simulink library "lib_lowphy"  (R2023b)
settings: Solver=VariableStepAuto  StartTime=0.0  StopTime=10.0  RelTol=1e-3
undefined symbols (not defined in the file or in its folder): AdvDSPBChannelOutDisplay, AdvDSPBDMemDisplay, AdvDSPBInDisplay, AdvDSPBOutDisplay, dpoly, dspba, dspba_ChannelInVis, dspba_ChannelOutVis, dspba_internal_get_channel_ports, evalAionMaskParam, fft_tb_in, ifft_tb_in, latency, latencyCorrection, max_FFTStages, max_NSubcarriers, primtype, UseDontCare, value
libraries: DSPBAPrim x637, DSPBAControl x55, $bdroot x16, DSPBAModelBus x12, DSPBAUtilities x6, DSPBABase x5, DSPBAWaveformSynth x4, DspbAdvFftLibrary x3, DSPBAVectorUtil x2, DspbAdvVfftPrefix x1
(part 2 of 9)

== system lib_lowphy/FFT_S2B/SignalProcessing ==
  fft_v_in : Inport
  cin : Inport  Port=2
  din : Inport  Port=3
  sync : Inport  Port=4
  nsc : Inport  Port=5
  size : Inport  Port=6
  SFNin : Inport  Port=7
  fft_gain_re : Inport  Port=8
  fft_gain_im : Inport  Port=9
  hcs_bypass : Inport  Port=10
  fft_shift : Inport  Port=11
  DC_SC_EN : Inport  Port=12
  ripple_comp_en : Inport  Port=13
  rc_bw_sel : Inport  Port=14
  eAxc : Inport  Port=15
  sym_metadata : Inport  Port=16
  BRandSCSelect1 : Subsystem  Opaque=on  mask(DSP Builder Advanced FFT Blockset){N=dspb_fft_multichannel.FFTsize, subchannels=dspb_fft_multichannel.subchannels}
      mask prompts: N "FFT Size"; subchannels "Number of subchannels (must be a power of 2)"
      mask help: Performs bit reversal of incoming FFT frames.
      mask init:
      | block = gcb;
      | 
      | % Check that we have a legal size
      | M = ceil(log2(N));
      | if not(N == 2^M)
      |     error('%s: %d is not a power of 2', block, N);
      | end
      | 
      | % Check that we have a legal number os subchannels
      | subchannelbits = ceil(log2(subchannels));
      | if not(subchannels == 2^subchannelbits)
      |     error('%s: subchannels count %d is not a power of 2', block, N);
      | end
      | 
      | % The permutation reverses the order of the address bits
      | bitrevperm = [M-1:-1:0];
      | 
      | % Prefix permutaion with unchanging subchannel bits
      | bitrevperm = [0:subchannelbits-1,bitrevperm+subchannelbits];
      | 
      | if 1 < subchannels
      |     subchannelString = sprintf('%d subchannels',subchannels);
      | else
      |     subchannelString = '';
      | end
      mask Help: helpview(dspba.GetHelp('BitReverseCore'));
      mask Display:
      | color('w');
      | image('dspba_fft.jpg');
      | port_label('input',1,'v');
      | port_label('input',2,'c');
      | port_label('input',3,'x');
      | port_label('input',4,'size');
      | port_label('input',5,'NSubCarr');
      | port_label('output',1,'qv');
      | port_label('output',2,'qc');
      | port_label('output',3,'q');
      | text(0.25, 0.8, 'Bit Reversal');
      | text(0.2, 0.7, 'and SubCarrier');
      | text(0.3, 0.6, 'Selection');
      | text(0.20,0.35,subchannelString);
  HCShift : Subsystem
  RXGainComp : Subsystem
  RXScaling : Subsystem
  Terminator : Terminator
  Terminator1 : Terminator
  Terminator2 : Terminator
  VFFT_btb : Subsystem  AncestorBlock=DspbAdvVfftPrefix/VFFT_btb  Opaque=on  mask{IFFT=dspb_fft_multichannel.IFFT, subchannels=dspb_fft_multichannel.subchannels, br_in=false, maxSize=dspb_fft_multichannel.maxsize, minSize=dspb_fft_multichannel.minsize, in_type=dspb_fft_multichannel.InputType, type_strings=dspba.fft.full_wordgrowth(true,false,11,fixdt(1,16,15),fixdt(1,18,17)), faithful=true}
      mask prompts: subchannels "Number of interleaved subchannels (must be a power of 2)"; br_in "Bit-reversed input"; maxSize "maxSize, where the (I)FFT has at most 2^maxSize points"; minSize "minSize, where the (I)FFT has at least 2^minSize points"; in_type "Input type"; type_strings "Twiddle/pruning specification"; faithful "Use faithful rounding"
      mask init:
      | block = gcb;
      | 
      | % Check that we have a legal number of subchannels
      | subchannelbits = ceil(log2(subchannels));
      | if not(subchannels == 2^subchannelbits)
      |     error('%s: subchannels count %d is not a power of 2', block, subchannels);
      | end
      | 
      | if IFFT
      |     FFTstring = 'IFFT';
      | else
      |     FFTstring = 'FFT';
      | end
      | 
      | if br_in
      |     directionString = 'BR->NAT';
      | else
      |     directionString = 'NAT->BR';
      | end
      | 
      | if 1 < subchannels
      |     subchannelString = sprintf('%d subchannels',subchannels);
      | else
      |     subchannelString = '';
      | end
      | 
      | % Largest number going into the VPD/VPM control inputs
      | maxBlocksizeBits = maxSize + subchannelbits;
      | 
      | % The width of the datapath needed to hold this number
      | adderWidth = ceil(log2(maxBlocksizeBits+1));
      mask Help: helpview(dspba.GetHelp('fft'));
      mask Display:
      | color('w');
      | image('dspba_fft.jpg');
      | port_label('input',1,'v');
      | port_label('input',2,'c');
      | port_label('input',3,'sop');
      | port_label('input',4,'size');
      | port_label('input',5,'d');
      | port_label('input',6,'nsc');
      | port_label('output',1,'qv');
      | port_label('output',2,'qc');
      | port_label('output',3,'qsop');
      | port_label('output',4,'qeop');
      | port_label('output',5,'qsize');
      | port_label('output',6,'q');
      | %text(0.25,0.75,sprintf('Cyclic Prefix'));
      | text(0.30,0.65,sprintf('V%s Core',FFTstring));
      | text(0.35,0.55,sprintf('2^{%d} to 2^{%d}',minSize,maxSize),'texmode','on');
      | text(0.30,0.45,directionString);
      | text(0.20,0.30,subchannelString);
      | text(0.25,0.20,sprintf('Back-To-Back'));
  rxnat_vout : Outport
  rxnat_chout : Outport  Port=2
  rxnat_dout : Outport  Port=3
  rx_time_out : Outport  Port=4
  td_fft_in_v : Outport  Port=5
  td_fft_in_ch : Outport  Port=6
  td_fft_in_d : Outport  Port=7
  nsc_out : Outport  Port=8
  size_out : Outport  Port=9
  td_time_out : Outport  Port=10
  fd_v : Outport  Port=11
  fd_c : Outport  Port=12
  fd_q : Outport  Port=13
  eAxC : Outport  Port=14
  metadata_sym_out : Outport  Port=15
  wires:
  BRandSCSelect1/6(eAxC_out) -> eAxC/1
  BRandSCSelect1/5(time_out) -> rx_time_out/1
  BRandSCSelect1/7(meatadata_sym_out) -> metadata_sym_out/1
  BRandSCSelect1/4(qsizeout) -> Terminator2/1
  BRandSCSelect1/1(qv) -> rxnat_vout/1  "rx_v_out"
  rc_bw_sel/1 -> BRandSCSelect1/9(rc_bw_sel)
  RXScaling/5(nsc_out) -> BRandSCSelect1/5(NSubCarr)
  ripple_comp_en/1 -> BRandSCSelect1/8(ripple_comp_en)
  RXScaling/4(size_out) -> BRandSCSelect1/4(FFTSize)
  RXScaling/3(dout) -> BRandSCSelect1/3(x), fd_q/1
  RXScaling/2(chout) -> fd_c/1, BRandSCSelect1/2(c)
  fft_shift/1 -> RXScaling/6(fft_shift)
  VFFT_btb/10(metadata_sym) -> RXScaling/9(sym_metadata)
  VFFT_btb/2(qc) -> RXScaling/2(chin)
  size/1 -> HCShift/5(size)
  RXGainComp/5(size_out) -> VFFT_btb/6(size), size_out/1
  HCShift/1(vout) -> RXGainComp/1(vin)
  RXScaling/1(vout) -> BRandSCSelect1/1(v), fd_v/1
  VFFT_btb/7(qnsc) -> RXScaling/5(nsc)
  HCShift/3(dout) -> RXGainComp/3(din)
  din/1 -> HCShift/3(din)
  hcs_bypass/1 -> HCShift/7(hcs_bypass)
  HCShift/6(SFNout) -> RXGainComp/8(time_in)
  RXGainComp/1(vout) -> VFFT_btb/1(v), VFFT_btb/3(sop), td_fft_in_v/1
  SFNin/1 -> HCShift/8(SFNin)
  VFFT_btb/1(qv) -> RXScaling/1(vin)
  BRandSCSelect1/2(qc) -> rxnat_chout/1
  VFFT_btb/3(qsop) -> Terminator/1
  sym_metadata/1 -> HCShift/10(sym_metadata)
  VFFT_btb/9(eAxC) -> RXScaling/8(eAxC)
  VFFT_btb/5(qsize) -> RXScaling/3(size)
  eAxc/1 -> HCShift/9(eAxC)
  nsc/1 -> HCShift/6(nsc)
  cin/1 -> HCShift/2(cin)
  RXScaling/7(eAxCout) -> BRandSCSelect1/10(eAxC)
  VFFT_btb/6(q) -> RXScaling/4(din)
  fft_v_in/1 -> HCShift/1(vin)
  RXGainComp/3(dout) -> td_fft_in_d/1, VFFT_btb/4(d)
  DC_SC_EN/1 -> BRandSCSelect1/7(DC_SC_EN)
  HCShift/2(cout) -> RXGainComp/2(chin)
  HCShift/4(nsc_out) -> RXGainComp/4(nsc)
  RXScaling/6(time_out) -> BRandSCSelect1/6(time_in)
  sync/1 -> HCShift/4(sync)
  HCShift/5(size_out) -> RXGainComp/5(size)
  RXGainComp/2(chout) -> td_fft_in_ch/1, VFFT_btb/2(c)
  VFFT_btb/8(time_out) -> RXScaling/7(time_in)
  RXGainComp/6(time_out) -> td_time_out/1, VFFT_btb/7(time_in)
  fft_gain_re/1 -> RXGainComp/6(fft_gain_re)
  HCShift/7(eAxC_out) -> RXGainComp/9(eAxC)
  HCShift/8(sym_metadataout) -> RXGainComp/10(sym_metadata)
  fft_gain_im/1 -> RXGainComp/7(fft_gain_im)
  BRandSCSelect1/3(q) -> rxnat_dout/1
  RXScaling/8(sym_metadataout) -> BRandSCSelect1/11(metadata_in)
  RXGainComp/7(eAxC_out) -> VFFT_btb/8(eAxC_no)
  VFFT_btb/4(qeop) -> Terminator1/1
  RXGainComp/4(nsc_out) -> nsc_out/1, VFFT_btb/5(nsc)
  RXGainComp/8(sym_metadata_out) -> VFFT_btb/9(sym_metadata)

== system lib_lowphy/PhaseCompensation/ComplexMixer ==
  note: mixer
  din1 : Inport
  vin : Inport  Port=2
  cin : Inport  Port=3
  sin : Inport  Port=4
  cos : Inport  Port=5
  Add : DSPBAPrim/Add  primtype=add  nInputs=evalAionMaskParam(gcb,'value',1)  nOutputs=1  omode=Inherit via internal rule with word growth  otype=sfix(16)  scale=2^-15  rndmethod=Unbiased  factor=1  satmethod=Symmetric  shift_vec=[0 1 2 -1]  value=2  inPortNames=[' '; ' ';]  outPortNames=[' ']  dspbaimage=dspba_prim.svg  text=fprintf('+');  style=Optimised  visibilities=1032+2^17+2^18+2^19  genFPC=off  floatRounding=correct  advOptions=[]  version=20211007
  Complex to Real-Imag1 : ComplexToRealImag
  ComplexMixer : DSPBAWaveformSynth/ComplexMixer  nInputRate=dspb_ifft_multichannel.ClockRate  nchan=1  nfreq=1  latency=6  simulationMode=Use Global Value  version=20090407
      settings: AttributesFormatString=%<latency>
  Const1 : DSPBAPrim/Const  primtype=const  nInputs=0  nOutputs=1  omode=Inherit via back propagation  otype=ufix(8)  scale=2^0  rndmethod=Unbiased  factor=1  satmethod=Symmetric  shift_vec=[0 1 2 -1]  value=1  inPortNames=['+'; '+';]  outPortNames=[' ']  dspbaimage=dspba_prim.svg  text=fprintf('%s', num2str(value));  style=Optimised  visibilities=8 + 1024  floatPrecision=float32_m23  warnSaturation=on  version=20211007  SampleTime=inf
  Mult : DSPBAPrim/Mult  primtype=mult  nInputs=2  nOutputs=1  omode=Inherit via internal rule  otype=sfix(16)  scale=2^-15  rndmethod=Unbiased  factor=1  satmethod=Symmetric  shift_vec=[0 1 2 -1]  value=0  inPortNames=[' '; ' ';]  outPortNames=[' ']  dspbaimage=dspba_prim.svg  text=fprintf('X');  style=Optimised  visibilities=8+2^18+2^19  floatPrecision=float32_m23  floatRounding=correct  advOptions=[]  version=20211007
  Mult1 : DSPBAPrim/Mult  primtype=mult  nInputs=2  nOutputs=1  omode=Inherit via internal rule  otype=sfix(16)  scale=2^-15  rndmethod=Unbiased  factor=1  satmethod=Symmetric  shift_vec=[0 1 2 -1]  value=0  inPortNames=[' '; ' ';]  outPortNames=[' ']  dspbaimage=dspba_prim.svg  text=fprintf('X');  style=Optimised  visibilities=8+2^18+2^19  floatPrecision=float32_m23  floatRounding=correct  advOptions=[]  version=20211007
  Real-Imag to Complex : RealImagToComplex
  Scalei : DSPBABase/Scale  otype=sfix(16)  scale=Op_frac_scaling  rndmethod=Biased  factor=1  satmethod=None  shift_vec=0  latency=1  simulationMode=Use Global Value  version=20130807
      settings: AttributesFormatString=%<latency>
  Scaleq : DSPBABase/Scale  otype=sfix(16)  scale=Op_frac_scaling  rndmethod=Biased  factor=1  satmethod=None  shift_vec=0  latency=1  simulationMode=Use Global Value  version=20130807
      settings: AttributesFormatString=%<latency>
  Scope : Scope
  Terminator{4..7} (4 alike) : Terminator
  dout1 : Outport
  vout : Outport  Port=2
  cout : Outport  Port=3
  wires:
  din1/1 -> Complex to Real-Imag1/1
  Scaleq/1 -> Real-Imag to Complex/2
  ComplexMixer/3 -> Scaleq/2, Scalei/2
  Scalei/1 -> Real-Imag to Complex/1
  Const1/1 -> Scaleq/4, Scalei/4
  Scaleq/3 -> Terminator7/1
  ComplexMixer/2 -> Scaleq/1
  Scaleq/2 -> Terminator6/1
  ComplexMixer/4 -> Scaleq/3, Scalei/3
  Complex to Real-Imag1/1 -> ComplexMixer/1
  Scalei/4 -> Terminator5/1
  Scaleq/4 -> Terminator4/1
  Complex to Real-Imag1/2 -> ComplexMixer/2
  ComplexMixer/1 -> Scalei/1
  Real-Imag to Complex/1 -> dout1/1
  sin/1 -> Mult/2, Mult/1, ComplexMixer/5
  vin/1 -> ComplexMixer/3
  cin/1 -> ComplexMixer/4
  cos/1 -> Mult1/2, Mult1/1, ComplexMixer/6
  Scalei/2 -> vout/1
  Scalei/3 -> cout/1
  Mult/1 -> Add/1
  Mult1/1 -> Add/2
  Add/1 -> Scope/1

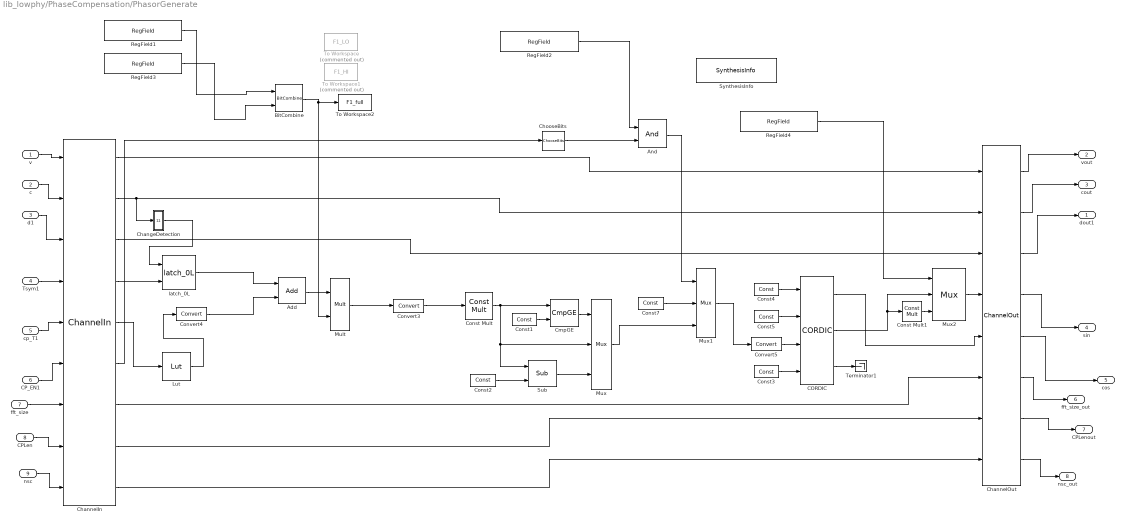
== system lib_lowphy/PhaseCompensation/PhasorGenerate ==
  v : Inport
  c : Inport  Port=2
  d1 : Inport  Port=3
  Tsym1 : Inport  Port=4
  cp_T1 : Inport  Port=5
  CP_EN1 : Inport  Port=6
  fft_size : Inport  Port=7
  CPLen : Inport  Port=8
  nsc : Inport  Port=9
  Add : DSPBAPrim/Add  primtype=add  nInputs=evalAionMaskParam(gcb,'value',1)  nOutputs=1  omode=Inherit via internal rule  otype=sfix(16)  scale=2^-15  rndmethod=Unbiased  factor=1  satmethod=Symmetric  shift_vec=[0 1 2 -1]  value=2  inPortNames=[' '; ' ';]  outPortNames=[' ']  dspbaimage=dspba_prim.svg  text=fprintf('+');  style=Optimised  visibilities=1032+2^17+2^18+2^19  genFPC=off  floatRounding=correct  advOptions=[]  version=20211007
  And : DSPBAPrim/And  primtype=and  nInputs=2  nOutputs=1  omode=Inherit via internal rule  otype=sfix(16)  scale=2^-15  rndmethod=Unbiased  factor=1  satmethod=Symmetric  shift_vec=[0 1 2 -1]  value=0  inPortNames=[' '; ' '; ' '; ' '; ' '; ' '; ' '; ' '; ' '; ' '; ' '; ' '; ' '; ' '; ' '; ' '; ]  outPortNames=[' ']  dspbaimage=dspba_prim.svg  text=fprintf('&');  style=Optimised  visibilities=8+2  version=20211007
  BitCombine : DSPBAPrim/BitCombine  primtype=bitcombine  nInputs=2  nOutputs=1  omode=Specify via dialog  otype=ufix(64)  scale=2^-56  rndmethod=Unbiased  factor=1  satmethod=Symmetric  shift_vec=[0 1 2 -1]  value=0  inPortNames=['l'; 'h';]  outPortNames=[' ']  dspbaimage=dspba_prim.svg  text=fprintf('[h,l]');  style=Optimised  visibilities=8+2  version=20211007
  CORDIC : DSPBAPrim/CORDIC  primtype=cordic  nInputs=4  nOutputs=3  omode=Inherit via internal rule  otype=sfix(16)  scale=2^-15  rndmethod=Unbiased  factor=1  satmethod=Symmetric  shift_vec=[0 1 2 -1]  value=0  inPortNames=['x'; 'y'; 'p'; 'v']  outPortNames=['x'; 'y'; 'p']  dspbaimage=dspba_prim_tall.svg  text=fprintf('cordic');  style=Optimised  visibilities=8  version=20211007
  ChangeDetection : Subsystem
  ChannelIn : DSPBAPrim/ChannelIn  primtype=channelin  nInputs=dspba_internal_get_channel_ports(gcb)  nOutputs=dspba_internal_get_channel_ports(gcb)  omode=Inherit via internal rule  otype=sfix(16)  scale=2^-15  rndmethod=Unbiased  factor=1  satmethod=Symmetric  shift_vec=[0 1 2 -1]  value=7  inPortNames=['v'; 'c'; '0'; '1'; '2'; '3'; '4'; '5'; '6'; '7'; '8'; '9'; 'A'; 'B'; 'D'; 'E'; 'F'; 'G'; 'H'; 'I'; 'J'; 'K'; 'L'; 'M'; 'N'; 'O'; 'P'; 'Q'; 'R'; 'S'; 'T'; 'U'; 'W'; 'X'; 'Y'; 'Z']  outPortNames=['v'; 'c'; '0'; '1'; '2'; '3'; '4'; '5'; '6'; '7'; '8'; '9'; 'A'; 'B'; 'D'; 'E'; 'F'; 'G'; 'H'; 'I'; 'J'; 'K'; 'L'; 'M'; 'N'; 'O'; 'P'; 'Q'; 'R'; 'S'; 'T'; 'U'; 'W'; 'X'; 'Y'; 'Z']  dspbaimage=dspba_prim_channel_tall.svg  text=fprintf('In');  style=Optimised  dataSignals=7  foldingEnabled=off  channels=1  sampleRate=200  packetBeginPresent=off  packetBeginEnabled=off  visibilities=dspba_ChannelInVis(gcb)  latencyCorrection=0  scheduleOrigin=on  version=20211214
  ChannelOut : DSPBAPrim/ChannelOut  primtype=channelout  nInputs=dspba_internal_get_channel_ports(gcb)  nOutputs=dspba_internal_get_channel_ports(gcb)  omode=Inherit via internal rule  otype=sfix(16)  scale=2^-15  rndmethod=Unbiased  factor=1  satmethod=Symmetric  shift_vec=[0 1 2 -1]  value=6  inPortNames=['v'; 'c'; '0'; '1'; '2'; '3'; '4'; '5'; '6'; '7'; '8'; '9'; 'A'; 'B'; 'D'; 'E'; 'F'; 'G'; 'H'; 'I'; 'J'; 'K'; 'L'; 'M'; 'N'; 'O'; 'P'; 'Q'; 'R'; 'S'; 'T'; 'U'; 'W'; 'X'; 'Y'; 'Z']  outPortNames=['v'; 'c'; '0'; '1'; '2'; '3'; '4'; '5'; '6'; '7'; '8'; '9'; 'A'; 'B'; 'D'; 'E'; 'F'; 'G'; 'H'; 'I'; 'J'; 'K'; 'L'; 'M'; 'N'; 'O'; 'P'; 'Q'; 'R'; 'S'; 'T'; 'U'; 'W'; 'X'; 'Y'; 'Z']  dspbaimage=dspba_prim_channel_tall.svg  text=fprintf('Out%s', AdvDSPBChannelOutDisplay(latency));  style=Optimised  dataSignals=6  foldingEnabled=off  channels=1  sampleRate=200  packetBeginPresent=off  packetBeginEnabled=off  visibilities=dspba_ChannelOutVis(gcb)  latency=38  latencyCorrection=0  version=20211214
  ChooseBits : DSPBAPrim/ChooseBits  primtype=choosebits  nInputs=1  nOutputs=1  omode=Inherit via internal rule  otype=fixdt(0,1,1)  scale=1  rndmethod=Unbiased  factor=1  satmethod=Symmetric  shift_vec=[0 1 2 -1]  value=[0]  inPortNames=[' '; ' ';]  outPortNames=[' ']  dspbaimage=dspba_prim.svg  text=fprintf('%s',dspba.perm2str(value));  style=Optimised  visibilities=1024  version=20211007
  CmpGE : DSPBAPrim/CmpGE  primtype=cmpgte  nInputs=2  nOutputs=1  omode=boolean  otype=sfix(16)  scale=2^-15  rndmethod=Unbiased  factor=1  satmethod=Symmetric  shift_vec=[0 1 2 -1]  value=0  inPortNames=['a'; 'b';]  outPortNames=[' ']  dspbaimage=dspba_prim.svg  text=fprintf('a>=b');  style=Optimised  visibilities=0  advOptions=[]  version=20211007
  Const Mult : DSPBAPrim/Const Mult  primtype=constmult  nInputs=1  nOutputs=1  omode=Specify via dialog  otype=sfix(16)  scale=2^-12  rndmethod=Unbiased  factor=1  satmethod=Symmetric  shift_vec=[0 1 2 -1]  value=2*pi  inPortNames=[' '; ' ';]  outPortNames=[' ']  dspbaimage=dspba_prim.svg  text=fprintf('cx');  style=Optimised  visibilities=8+2^10+2^17+2^18  floatRounding=correct  advOptions=[]  version=20211007
  Const Mult1 : DSPBAPrim/Const Mult  primtype=constmult  nInputs=1  nOutputs=1  omode=Specify via dialog  otype=sfix(16)  scale=2^-12  rndmethod=Unbiased  factor=1  satmethod=Symmetric  shift_vec=[0 1 2 -1]  value=-1  inPortNames=[' '; ' ';]  outPortNames=[' ']  dspbaimage=dspba_prim.svg  text=fprintf('cx');  style=Optimised  visibilities=8+2^10+2^17+2^18  floatRounding=correct  advOptions=[]  version=20211007
  Const1 : DSPBAPrim/Const  primtype=const  nInputs=0  nOutputs=1  omode=Specify via dialog  otype=sfix(16)  scale=2^-12  rndmethod=Unbiased  factor=1  satmethod=Symmetric  shift_vec=[0 1 2 -1]  value=pi  inPortNames=['+'; '+';]  outPortNames=[' ']  dspbaimage=dspba_prim.svg  text=fprintf('%s', num2str(value));  style=Optimised  visibilities=8 + 1024  floatPrecision=float32_m23  warnSaturation=on  version=20211007  SampleTime=inf
  Const2 : DSPBAPrim/Const  primtype=const  nInputs=0  nOutputs=1  omode=Specify via dialog  otype=sfix(16)  scale=2^-12  rndmethod=Unbiased  factor=1  satmethod=Symmetric  shift_vec=[0 1 2 -1]  value=2*pi  inPortNames=['+'; '+';]  outPortNames=[' ']  dspbaimage=dspba_prim.svg  text=fprintf('%s', num2str(value));  style=Optimised  visibilities=8 + 1024  floatPrecision=float32_m23  warnSaturation=on  version=20211007  SampleTime=inf
  Const3 : DSPBAPrim/Const  primtype=const  nInputs=0  nOutputs=1  omode=boolean  otype=sfix(16)  scale=2^-12  rndmethod=Unbiased  factor=1  satmethod=Symmetric  shift_vec=[0 1 2 -1]  value=0  inPortNames=['+'; '+';]  outPortNames=[' ']  dspbaimage=dspba_prim.svg  text=fprintf('%s', num2str(value));  style=Optimised  visibilities=8 + 1024  floatPrecision=float32_m23  warnSaturation=on  version=20211007  SampleTime=inf
  Const4 : DSPBAPrim/Const  primtype=const  nInputs=0  nOutputs=1  omode=Specify via dialog  otype=sfix(16)  scale=2^-15  rndmethod=Unbiased  factor=1  satmethod=Symmetric  shift_vec=[0 1 2 -1]  value=1/cordic_gain  inPortNames=['+'; '+';]  outPortNames=[' ']  dspbaimage=dspba_prim.svg  text=fprintf('%s', num2str(value));  style=Optimised  visibilities=8 + 1024  floatPrecision=float32_m23  warnSaturation=on  version=20211007  SampleTime=inf
  Const5 : DSPBAPrim/Const  primtype=const  nInputs=0  nOutputs=1  omode=Specify via dialog  otype=sfix(16)  scale=2^-15  rndmethod=Unbiased  factor=1  satmethod=Symmetric  shift_vec=[0 1 2 -1]  value=0  inPortNames=['+'; '+';]  outPortNames=[' ']  dspbaimage=dspba_prim.svg  text=fprintf('%s', num2str(value));  style=Optimised  visibilities=8 + 1024  floatPrecision=float32_m23  warnSaturation=on  version=20211007  SampleTime=inf
  Const7 : DSPBAPrim/Const  primtype=const  nInputs=0  nOutputs=1  omode=Specify via dialog  otype=sfix(16)  scale=2^-15  rndmethod=Unbiased  factor=1  satmethod=Symmetric  shift_vec=[0 1 2 -1]  value=0  inPortNames=['+'; '+';]  outPortNames=[' ']  dspbaimage=dspba_prim.svg  text=fprintf('%s', num2str(value));  style=Optimised  visibilities=8 + 1024  floatPrecision=float32_m23  warnSaturation=on  version=20211007  SampleTime=inf
  Convert3 : DSPBAPrim/Convert  primtype=convert  nInputs=1  nOutputs=1  omode=Specify via dialog  otype=ufix(16)  scale=2^-16  rndmethod=Biased  factor=1  satmethod=None  shift_vec=[0 1 2 -1]  value=round([0:255]/17)  inPortNames=[' '; ' ';]  outPortNames=[' '; 'c']  dspbaimage=dspba_prim_wide.svg  text=fprintf('convert');  style=Optimised  visibilities=8+64+256+2^17  clipdetect=off  floatPrecision=float32_m23  advOptions=[]  version=20211007
  Convert4 : DSPBAPrim/Convert  primtype=convert  nInputs=1  nOutputs=1  omode=Specify via dialog  otype=ufix(32)  scale=2^-18  rndmethod=Biased  factor=1  satmethod=None  shift_vec=[0 1 2 -1]  value=round([0:255]/17)  inPortNames=[' '; ' ';]  outPortNames=[' '; 'c']  dspbaimage=dspba_prim_wide.svg  text=fprintf('convert');  style=Optimised  visibilities=8+64+256+2^17  clipdetect=off  floatPrecision=float32_m23  advOptions=[]  version=20211007
  Convert5 : DSPBAPrim/Convert  primtype=convert  nInputs=1  nOutputs=1  omode=Specify via dialog  otype=sfix(16)  scale=2^-13  rndmethod=Biased  factor=1  satmethod=None  shift_vec=[0 1 2 -1]  value=round([0:255]/17)  inPortNames=[' '; ' ';]  outPortNames=[' '; 'c']  dspbaimage=dspba_prim_wide.svg  text=fprintf('convert');  style=Optimised  visibilities=8+64+256+2^17  clipdetect=off  floatPrecision=float32_m23  advOptions=[]  version=20211007
  Lut : DSPBAPrim/Lut  primtype=lut  nInputs=1  nOutputs=1  omode=Inherit via internal rule  otype=sfix(16)  scale=2^-15  rndmethod=Unbiased  factor=1  satmethod=Symmetric  shift_vec=[0 1 2 -1]  value=CPSample_Vector_LUT  inPortNames=[' '; ' ';]  outPortNames=[' ']  dspbaimage=dspba_prim.svg  text=fprintf('LUT');  style=Optimised  visibilities=8 + 1024  floatPrecision=float32_m23  version=20211007
  Mult : DSPBAPrim/Mult  primtype=mult  nInputs=2  nOutputs=1  omode=Inherit via internal rule  otype=sfix(16)  scale=2^-15  rndmethod=Unbiased  factor=1  satmethod=Symmetric  shift_vec=[0 1 2 -1]  value=0  inPortNames=[' '; ' ';]  outPortNames=[' ']  dspbaimage=dspba_prim.svg  text=fprintf('X');  style=Optimised  visibilities=8+2^18+2^19  floatPrecision=float64_m52  floatRounding=correct  advOptions=[]  version=20211007
  Mux : DSPBAPrim/Mux  primtype=mux  nInputs=evalAionMaskParam(gcb,'value',1)+1  nOutputs=1  omode=Inherit via internal rule  otype=sfix(16)  scale=2^-15  rndmethod=Unbiased  factor=1  satmethod=Symmetric  shift_vec=[0 1 2 -1]  value=2  inPortNames=['s '; 'd0'; 'd1'; 'd2'; 'd3'; 'd4'; 'd5'; 'd6'; 'd7'; 'd8'; 'd9';]  outPortNames=[' ']  dspbaimage=dspba_prim_tall.svg  text=fprintf('%s', primtype);  style=Optimised  visibilities=1032  version=20211007
  Mux1 : DSPBAPrim/Mux  primtype=mux  nInputs=evalAionMaskParam(gcb,'value',1)+1  nOutputs=1  omode=Inherit via internal rule  otype=sfix(16)  scale=2^-15  rndmethod=Unbiased  factor=1  satmethod=Symmetric  shift_vec=[0 1 2 -1]  value=2  inPortNames=['s '; 'd0'; 'd1'; 'd2'; 'd3'; 'd4'; 'd5'; 'd6'; 'd7'; 'd8'; 'd9';]  outPortNames=[' ']  dspbaimage=dspba_prim_tall.svg  text=fprintf('%s', primtype);  style=Optimised  visibilities=1032  version=20211007
  Mux2 : DSPBAPrim/Mux  primtype=mux  nInputs=evalAionMaskParam(gcb,'value',1)+1  nOutputs=1  omode=Specify via dialog  otype=sfix(18)  scale=2^-15  rndmethod=Unbiased  factor=1  satmethod=Symmetric  shift_vec=[0 1 2 -1]  value=2  inPortNames=['s '; 'd0'; 'd1'; 'd2'; 'd3'; 'd4'; 'd5'; 'd6'; 'd7'; 'd8'; 'd9';]  outPortNames=[' ']  dspbaimage=dspba_prim_tall.svg  text=fprintf('%s', primtype);  style=Optimised  visibilities=1032  version=20211007
  RegField1 : DSPBAModelBus/RegField  reg_name=MMoffset.F1_regLSB  reg_rwmode=Read/Write  reg_msb=31  reg_lsb=0  reg_mode=Specify via dialog  reg_type=ufix(32)  reg_scale=2^0  reg_init=F1_LSB  reg_desc=32 bit LSB of Carrier Center Frequency  reg_modal=off  reg_desc0=0  reg_desc1=0  reg_desc2=0  reg_desc3=0  reg_desc4=0  reg_desc5=0  reg_desc6=0  reg_desc7=0  reg_addr=0  SampleTime=-1  version=20090407
  RegField2 : DSPBAModelBus/RegField  reg_name=MMoffset.Enable_reg1  reg_rwmode=Read/Write  reg_msb=0  reg_lsb=0  reg_mode=Specify via dialog  reg_type=ufix(1)  reg_scale=2^0  reg_init=1  reg_desc=Enable/Disable Phase Compensation  reg_modal=off  reg_desc0=0  reg_desc1=0  reg_desc2=0  reg_desc3=0  reg_desc4=0  reg_desc5=0  reg_desc6=0  reg_desc7=0  reg_addr=2  SampleTime=-1  version=20090407
  RegField3 : DSPBAModelBus/RegField  reg_name=MMoffset.F1_regMSB  reg_rwmode=Read/Write  reg_msb=31  reg_lsb=0  reg_mode=Specify via dialog  reg_type=ufix(32)  reg_scale=2^0  reg_init=F1_MSB  reg_desc=32 bit MSB of Carrier Center Frequency  reg_modal=off  reg_desc0=0  reg_desc1=0  reg_desc2=0  reg_desc3=0  reg_desc4=0  reg_desc5=0  reg_desc6=0  reg_desc7=0  reg_addr=1  SampleTime=-1  version=20090407
  RegField4 : DSPBAModelBus/RegField  reg_name=MMoffset.PhaseGen_reg  reg_rwmode=Read/Write  reg_msb=0  reg_lsb=0  reg_mode=Specify via dialog  reg_type=ufix(1)  reg_scale=2^0  reg_init=PhaseGen_TXRX  reg_desc=Enable/Disable Phase Compensation  reg_modal=off  reg_desc0=0  reg_desc1=0  reg_desc2=0  reg_desc3=0  reg_desc4=0  reg_desc5=0  reg_desc6=0  reg_desc7=0  reg_addr=3  SampleTime=-1  version=20090407
  Sub : DSPBAPrim/Sub  primtype=sub  nInputs=2  nOutputs=1  omode=Inherit via internal rule with word growth  otype=sfix(16)  scale=2^-15  rndmethod=Unbiased  factor=1  satmethod=Symmetric  shift_vec=[0 1 2 -1]  value=0  inPortNames=['+'; '-';]  outPortNames=[' ']  dspbaimage=dspba_prim.svg  text=fprintf('-');  style=Optimised  visibilities=8+2^17+2^18  floatRounding=correct  advOptions=[]  version=20211007
  SynthesisInfo : DSPBAPrim/SynthesisInfo  primtype=synthinfo  nInputs=0  nOutputs=0  omode=Inherit via internal rule  otype=sfix(16)  scale=2^-15  rndmethod=Truncate  factor=1  satmethod=Symmetric  shift_vec=[0 1 2 -1]  value=99  inPortNames=[' '; ' ';]  outPortNames=[' ']  dspbaimage=dspba_prim_ctrl.jpg  text=fprintf('Style=%s', style);  style=Scheduled  visibilities=2^17+2^18+2^19+2^20+2^21+2^22+2^23+2^24  constraintPair=None  constraintRelation=>  constraintLimit=2  modelRefSign=+  modelRef=''  showSchedule=off  simulationMode=Use Global Value  resetMinimization=Conditional - On for ChannelIn/Out only  version=20220106
  Terminator1 : Terminator
  To Workspace : ToWorkspace  Commented=on  VariableName=F1_LO  SampleTime=-1
  To Workspace1 : ToWorkspace  Commented=on  VariableName=F1_HI  SampleTime=-1
  To Workspace2 : ToWorkspace  VariableName=F1_full  SampleTime=-1
  latch_0L : DSPBAControl/latch_0L
  dout1 : Outport
  vout : Outport  Port=2
  cout : Outport  Port=3
  sin : Outport  Port=4
  cos : Outport  Port=5
  fft_size_out : Outport  Port=6
  CPLenout : Outport  Port=7
  nsc_out : Outport  Port=8
  wires:
  c/1 -> ChannelIn/2
  ChannelIn/1 -> ChannelOut/1
  ChannelIn/2 -> ChangeDetection/1(In1), ChannelOut/2
  v/1 -> ChannelIn/1
  ChannelIn/3 -> ChannelOut/3
  d1/1 -> ChannelIn/3
  ChannelOut/1 -> vout/1
  ChannelOut/2 -> cout/1
  ChannelOut/3 -> dout1/1
  ChannelOut/4 -> sin/1
  ChannelIn/5 -> Lut/1
  Convert3/1 -> Const Mult/1
  Const Mult/1 -> Sub/1, Mux/2, CmpGE/1
  Const1/1 -> CmpGE/2
  CmpGE/1 -> Mux/1
  Sub/1 -> Mux/3
  Const2/1 -> Sub/2
  Const3/1 -> CORDIC/4
  Const4/1 -> CORDIC/1
  Const5/1 -> CORDIC/2
  CORDIC/3 -> Terminator1/1
  Convert5/1 -> CORDIC/3
  ChannelOut/5 -> cos/1
  RegField2/1 -> And/1
  Const7/1 -> Mux1/2
  CORDIC/1 -> ChannelOut/5
  Mux1/1 -> Convert5/1
  Lut/1 -> Convert4/1
  Mult/1 -> Convert3/1
  Mux/1 -> Mux1/3
  Add/1 -> Mult/1
  Convert4/1 -> Add/2
  ChannelIn/6 -> ChooseBits/1
  And/1 -> Mux1/1
  ChooseBits/1 -> And/2
  BitCombine/1 -> Mult/2, To Workspace2/1
  Tsym1/1 -> ChannelIn/4
  cp_T1/1 -> ChannelIn/5
  CP_EN1/1 -> ChannelIn/6
  RegField3/1 -> BitCombine/2
  RegField1/1 -> BitCombine/1
  fft_size/1 -> ChannelIn/7
  CPLen/1 -> ChannelIn/8
  nsc/1 -> ChannelIn/9
  ChannelOut/6 -> fft_size_out/1
  ChannelOut/7 -> CPLenout/1
  ChannelOut/8 -> nsc_out/1
  ChannelIn/7 -> ChannelOut/6
  ChannelIn/8 -> ChannelOut/7
  ChannelIn/9 -> ChannelOut/8
  latch_0L/1 -> Add/1
  ChangeDetection/1(Out1) -> latch_0L/1
  ChannelIn/4 -> latch_0L/2
  Mux2/1 -> ChannelOut/4
  CORDIC/2 -> Const Mult1/1, Mux2/2
  Const Mult1/1 -> Mux2/3
  RegField4/1 -> Mux2/1

== system lib_lowphy/PhaseCompensation_lite/ComplexMixer ==
  note: mixer
  din1 : Inport
  vin : Inport  Port=2
  cin : Inport  Port=3
  sin : Inport  Port=4
  cos : Inport  Port=5
  Add : DSPBAPrim/Add  primtype=add  nInputs=evalAionMaskParam(gcb,'value',1)  nOutputs=1  omode=Inherit via internal rule with word growth  otype=sfix(16)  scale=2^-15  rndmethod=Unbiased  factor=1  satmethod=Symmetric  shift_vec=[0 1 2 -1]  value=2  inPortNames=[' '; ' ';]  outPortNames=[' ']  dspbaimage=dspba_prim.svg  text=fprintf('+');  style=Optimised  visibilities=1032+2^17+2^18+2^19  genFPC=off  floatRounding=correct  advOptions=[]  version=20211007
  Complex to Real-Imag1 : ComplexToRealImag
  ComplexMixer : DSPBAWaveformSynth/ComplexMixer  nInputRate=dspb_ifft_multichannel.ClockRate  nchan=1  nfreq=1  latency=6  simulationMode=Use Global Value  version=20090407
      settings: AttributesFormatString=%<latency>
  Const1 : DSPBAPrim/Const  primtype=const  nInputs=0  nOutputs=1  omode=Inherit via back propagation  otype=ufix(8)  scale=2^0  rndmethod=Unbiased  factor=1  satmethod=Symmetric  shift_vec=[0 1 2 -1]  value=1  inPortNames=['+'; '+';]  outPortNames=[' ']  dspbaimage=dspba_prim.svg  text=fprintf('%s', num2str(value));  style=Optimised  visibilities=8 + 1024  floatPrecision=float32_m23  warnSaturation=on  version=20211007  SampleTime=inf
  Mult : DSPBAPrim/Mult  primtype=mult  nInputs=2  nOutputs=1  omode=Inherit via internal rule  otype=sfix(16)  scale=2^-15  rndmethod=Unbiased  factor=1  satmethod=Symmetric  shift_vec=[0 1 2 -1]  value=0  inPortNames=[' '; ' ';]  outPortNames=[' ']  dspbaimage=dspba_prim.svg  text=fprintf('X');  style=Optimised  visibilities=8+2^18+2^19  floatPrecision=float32_m23  floatRounding=correct  advOptions=[]  version=20211007
  Mult1 : DSPBAPrim/Mult  primtype=mult  nInputs=2  nOutputs=1  omode=Inherit via internal rule  otype=sfix(16)  scale=2^-15  rndmethod=Unbiased  factor=1  satmethod=Symmetric  shift_vec=[0 1 2 -1]  value=0  inPortNames=[' '; ' ';]  outPortNames=[' ']  dspbaimage=dspba_prim.svg  text=fprintf('X');  style=Optimised  visibilities=8+2^18+2^19  floatPrecision=float32_m23  floatRounding=correct  advOptions=[]  version=20211007
  Real-Imag to Complex : RealImagToComplex
  Scalei : DSPBABase/Scale  otype=sfix(16)  scale=Op_frac_scaling  rndmethod=Biased  factor=1  satmethod=None  shift_vec=0  latency=1  simulationMode=Use Global Value  version=20130807
      settings: AttributesFormatString=%<latency>
  Scaleq : DSPBABase/Scale  otype=sfix(16)  scale=Op_frac_scaling  rndmethod=Biased  factor=1  satmethod=None  shift_vec=0  latency=1  simulationMode=Use Global Value  version=20130807
      settings: AttributesFormatString=%<latency>
  Scope : Scope
  Terminator{4..7} (4 alike) : Terminator
  dout1 : Outport
  vout : Outport  Port=2
  cout : Outport  Port=3
  wires:
  din1/1 -> Complex to Real-Imag1/1
  Scaleq/1 -> Real-Imag to Complex/2
  ComplexMixer/3 -> Scaleq/2, Scalei/2
  Scalei/1 -> Real-Imag to Complex/1
  Const1/1 -> Scaleq/4, Scalei/4
  Scaleq/3 -> Terminator7/1
  ComplexMixer/2 -> Scaleq/1
  Scaleq/2 -> Terminator6/1
  ComplexMixer/4 -> Scaleq/3, Scalei/3
  Complex to Real-Imag1/1 -> ComplexMixer/1
  Scalei/4 -> Terminator5/1
  Scaleq/4 -> Terminator4/1
  Complex to Real-Imag1/2 -> ComplexMixer/2
  ComplexMixer/1 -> Scalei/1
  Real-Imag to Complex/1 -> dout1/1
  sin/1 -> Mult/2, Mult/1, ComplexMixer/5
  vin/1 -> ComplexMixer/3
  cin/1 -> ComplexMixer/4
  cos/1 -> Mult1/2, Mult1/1, ComplexMixer/6
  Scalei/2 -> vout/1
  Scalei/3 -> cout/1
  Mult/1 -> Add/1
  Mult1/1 -> Add/2
  Add/1 -> Scope/1

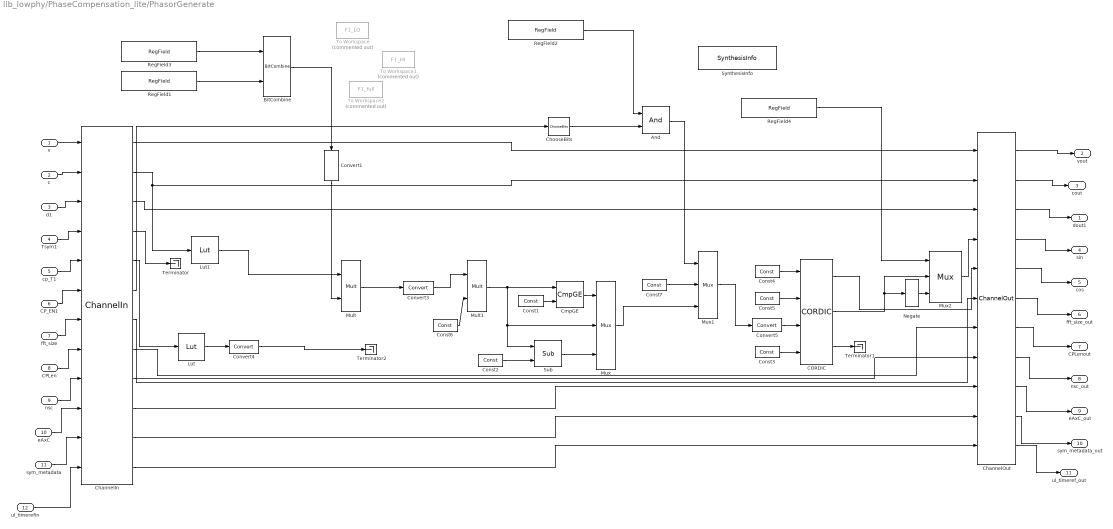
== system lib_lowphy/PhaseCompensation_lite/PhasorGenerate ==
  v : Inport
  c : Inport  Port=2
  d1 : Inport  Port=3
  Tsym1 : Inport  Port=4
  cp_T1 : Inport  Port=5
  CP_EN1 : Inport  Port=6
  fft_size : Inport  Port=7
  CPLen : Inport  Port=8
  nsc : Inport  Port=9
  eAxC : Inport  Port=10
  sym_metadata : Inport  Port=11
  ul_timerefin : Inport  Port=12
  And : DSPBAPrim/And  primtype=and  nInputs=2  nOutputs=1  omode=Inherit via internal rule  otype=sfix(16)  scale=2^-15  rndmethod=Unbiased  factor=1  satmethod=Symmetric  shift_vec=[0 1 2 -1]  value=0  inPortNames=[' '; ' '; ' '; ' '; ' '; ' '; ' '; ' '; ' '; ' '; ' '; ' '; ' '; ' '; ' '; ' '; ]  outPortNames=[' ']  dspbaimage=dspba_prim.svg  text=fprintf('&');  style=Optimised  visibilities=8+2  version=20211007
  BitCombine : DSPBAPrim/BitCombine  primtype=bitcombine  nInputs=2  nOutputs=1  omode=Specify via dialog  otype=ufix(64)  scale=2^-32  rndmethod=Unbiased  factor=1  satmethod=Symmetric  shift_vec=[0 1 2 -1]  value=0  inPortNames=['l'; 'h';]  outPortNames=[' ']  dspbaimage=dspba_prim.svg  text=fprintf('[h,l]');  style=Optimised  visibilities=8+2  version=20211007
  CORDIC : DSPBAPrim/CORDIC  primtype=cordic  nInputs=4  nOutputs=3  omode=Inherit via internal rule  otype=sfix(16)  scale=2^-15  rndmethod=Unbiased  factor=1  satmethod=Symmetric  shift_vec=[0 1 2 -1]  value=0  inPortNames=['x'; 'y'; 'p'; 'v']  outPortNames=['x'; 'y'; 'p']  dspbaimage=dspba_prim_tall.svg  text=fprintf('cordic');  style=Optimised  visibilities=8  version=20211007
  ChannelIn : DSPBAPrim/ChannelIn  primtype=channelin  nInputs=dspba_internal_get_channel_ports(gcb)  nOutputs=dspba_internal_get_channel_ports(gcb)  omode=Inherit via internal rule  otype=sfix(16)  scale=2^-15  rndmethod=Unbiased  factor=1  satmethod=Symmetric  shift_vec=[0 1 2 -1]  value=10  inPortNames=['v'; 'c'; '0'; '1'; '2'; '3'; '4'; '5'; '6'; '7'; '8'; '9'; 'A'; 'B'; 'D'; 'E'; 'F'; 'G'; 'H'; 'I'; 'J'; 'K'; 'L'; 'M'; 'N'; 'O'; 'P'; 'Q'; 'R'; 'S'; 'T'; 'U'; 'W'; 'X'; 'Y'; 'Z']  outPortNames=['v'; 'c'; '0'; '1'; '2'; '3'; '4'; '5'; '6'; '7'; '8'; '9'; 'A'; 'B'; 'D'; 'E'; 'F'; 'G'; 'H'; 'I'; 'J'; 'K'; 'L'; 'M'; 'N'; 'O'; 'P'; 'Q'; 'R'; 'S'; 'T'; 'U'; 'W'; 'X'; 'Y'; 'Z']  dspbaimage=dspba_prim_channel_tall.svg  text=fprintf('In');  style=Optimised  dataSignals=10  foldingEnabled=off  channels=1  sampleRate=200  packetBeginPresent=off  packetBeginEnabled=off  visibilities=dspba_ChannelInVis(gcb)  latencyCorrection=0  scheduleOrigin=on  version=20211214
  ChannelOut : DSPBAPrim/ChannelOut  primtype=channelout  nInputs=dspba_internal_get_channel_ports(gcb)  nOutputs=dspba_internal_get_channel_ports(gcb)  omode=Inherit via internal rule  otype=sfix(16)  scale=2^-15  rndmethod=Unbiased  factor=1  satmethod=Symmetric  shift_vec=[0 1 2 -1]  value=9  inPortNames=['v'; 'c'; '0'; '1'; '2'; '3'; '4'; '5'; '6'; '7'; '8'; '9'; 'A'; 'B'; 'D'; 'E'; 'F'; 'G'; 'H'; 'I'; 'J'; 'K'; 'L'; 'M'; 'N'; 'O'; 'P'; 'Q'; 'R'; 'S'; 'T'; 'U'; 'W'; 'X'; 'Y'; 'Z']  outPortNames=['v'; 'c'; '0'; '1'; '2'; '3'; '4'; '5'; '6'; '7'; '8'; '9'; 'A'; 'B'; 'D'; 'E'; 'F'; 'G'; 'H'; 'I'; 'J'; 'K'; 'L'; 'M'; 'N'; 'O'; 'P'; 'Q'; 'R'; 'S'; 'T'; 'U'; 'W'; 'X'; 'Y'; 'Z']  dspbaimage=dspba_prim_channel_tall.svg  text=fprintf('Out%s', AdvDSPBChannelOutDisplay(latency));  style=Optimised  dataSignals=9  foldingEnabled=off  channels=1  sampleRate=200  packetBeginPresent=off  packetBeginEnabled=off  visibilities=dspba_ChannelOutVis(gcb)  latency=38  latencyCorrection=0  version=20211214
  ChooseBits : DSPBAPrim/ChooseBits  primtype=choosebits  nInputs=1  nOutputs=1  omode=Inherit via internal rule  otype=fixdt(0,1,1)  scale=1  rndmethod=Unbiased  factor=1  satmethod=Symmetric  shift_vec=[0 1 2 -1]  value=[0]  inPortNames=[' '; ' ';]  outPortNames=[' ']  dspbaimage=dspba_prim.svg  text=fprintf('%s',dspba.perm2str(value));  style=Optimised  visibilities=1024  version=20211007
  CmpGE : DSPBAPrim/CmpGE  primtype=cmpgte  nInputs=2  nOutputs=1  omode=boolean  otype=sfix(16)  scale=2^-15  rndmethod=Unbiased  factor=1  satmethod=Symmetric  shift_vec=[0 1 2 -1]  value=0  inPortNames=['a'; 'b';]  outPortNames=[' ']  dspbaimage=dspba_prim.svg  text=fprintf('a>=b');  style=Optimised  visibilities=0  advOptions=[]  version=20211007
  Const1 : DSPBAPrim/Const  primtype=const  nInputs=0  nOutputs=1  omode=Specify via dialog  otype=sfix(16)  scale=2^-12  rndmethod=Unbiased  factor=1  satmethod=Symmetric  shift_vec=[0 1 2 -1]  value=pi  inPortNames=['+'; '+';]  outPortNames=[' ']  dspbaimage=dspba_prim.svg  text=fprintf('%s', num2str(value));  style=Optimised  visibilities=8 + 1024  floatPrecision=float32_m23  warnSaturation=on  version=20211007  SampleTime=inf
  Const2 : DSPBAPrim/Const  primtype=const  nInputs=0  nOutputs=1  omode=Specify via dialog  otype=sfix(16)  scale=2^-12  rndmethod=Unbiased  factor=1  satmethod=Symmetric  shift_vec=[0 1 2 -1]  value=2*pi  inPortNames=['+'; '+';]  outPortNames=[' ']  dspbaimage=dspba_prim.svg  text=fprintf('%s', num2str(value));  style=Optimised  visibilities=8 + 1024  floatPrecision=float32_m23  warnSaturation=on  version=20211007  SampleTime=inf
  Const3 : DSPBAPrim/Const  primtype=const  nInputs=0  nOutputs=1  omode=boolean  otype=sfix(16)  scale=2^-12  rndmethod=Unbiased  factor=1  satmethod=Symmetric  shift_vec=[0 1 2 -1]  value=0  inPortNames=['+'; '+';]  outPortNames=[' ']  dspbaimage=dspba_prim.svg  text=fprintf('%s', num2str(value));  style=Optimised  visibilities=8 + 1024  floatPrecision=float32_m23  warnSaturation=on  version=20211007  SampleTime=inf
  Const4 : DSPBAPrim/Const  primtype=const  nInputs=0  nOutputs=1  omode=Specify via dialog  otype=sfix(16)  scale=2^-15  rndmethod=Unbiased  factor=1  satmethod=Symmetric  shift_vec=[0 1 2 -1]  value=1/cordic_gain  inPortNames=['+'; '+';]  outPortNames=[' ']  dspbaimage=dspba_prim.svg  text=fprintf('%s', num2str(value));  style=Optimised  visibilities=8 + 1024  floatPrecision=float32_m23  warnSaturation=on  version=20211007  SampleTime=inf
  Const5 : DSPBAPrim/Const  primtype=const  nInputs=0  nOutputs=1  omode=Specify via dialog  otype=sfix(16)  scale=2^-15  rndmethod=Unbiased  factor=1  satmethod=Symmetric  shift_vec=[0 1 2 -1]  value=0  inPortNames=['+'; '+';]  outPortNames=[' ']  dspbaimage=dspba_prim.svg  text=fprintf('%s', num2str(value));  style=Optimised  visibilities=8 + 1024  floatPrecision=float32_m23  warnSaturation=on  version=20211007  SampleTime=inf
  Const6 : DSPBAPrim/Const  primtype=const  nInputs=0  nOutputs=1  omode=Specify via dialog  otype=sfix(16)  scale=2^-12  rndmethod=Unbiased  factor=1  satmethod=Symmetric  shift_vec=[0 1 2 -1]  value=2*pi  inPortNames=['+'; '+';]  outPortNames=[' ']  dspbaimage=dspba_prim.svg  text=fprintf('%s', num2str(value));  style=Optimised  visibilities=8 + 1024  floatPrecision=float32_m23  warnSaturation=on  version=20211007  SampleTime=inf
  Const7 : DSPBAPrim/Const  primtype=const  nInputs=0  nOutputs=1  omode=Specify via dialog  otype=sfix(16)  scale=2^-15  rndmethod=Unbiased  factor=1  satmethod=Symmetric  shift_vec=[0 1 2 -1]  value=0  inPortNames=['+'; '+';]  outPortNames=[' ']  dspbaimage=dspba_prim.svg  text=fprintf('%s', num2str(value));  style=Optimised  visibilities=8 + 1024  floatPrecision=float32_m23  warnSaturation=on  version=20211007  SampleTime=inf
  Convert1 : DSPBAPrim/Convert  primtype=convert  nInputs=1  nOutputs=1  omode=Specify via dialog  otype=ufix(40)  scale=2^-32  rndmethod=Biased  factor=1  satmethod=None  shift_vec=[0 1 2 -1]  value=round([0:255]/17)  inPortNames=[' '; ' ';]  outPortNames=[' '; 'c']  dspbaimage=dspba_prim_wide.svg  text=fprintf('convert');  style=Optimised  visibilities=8+64+256+2^17  clipdetect=off  floatPrecision=float32_m23  advOptions=[]  version=20211007
  Convert3 : DSPBAPrim/Convert  primtype=convert  nInputs=1  nOutputs=1  omode=Specify via dialog  otype=ufix(16)  scale=2^-16  rndmethod=Biased  factor=1  satmethod=None  shift_vec=[0 1 2 -1]  value=round([0:255]/17)  inPortNames=[' '; ' ';]  outPortNames=[' '; 'c']  dspbaimage=dspba_prim_wide.svg  text=fprintf('convert');  style=Optimised  visibilities=8+64+256+2^17  clipdetect=off  floatPrecision=float32_m23  advOptions=[]  version=20211007
  Convert4 : DSPBAPrim/Convert  primtype=convert  nInputs=1  nOutputs=1  omode=Specify via dialog  otype=ufix(32)  scale=2^-18  rndmethod=Biased  factor=1  satmethod=None  shift_vec=[0 1 2 -1]  value=round([0:255]/17)  inPortNames=[' '; ' ';]  outPortNames=[' '; 'c']  dspbaimage=dspba_prim_wide.svg  text=fprintf('convert');  style=Optimised  visibilities=8+64+256+2^17  clipdetect=off  floatPrecision=float32_m23  advOptions=[]  version=20211007
  Convert5 : DSPBAPrim/Convert  primtype=convert  nInputs=1  nOutputs=1  omode=Specify via dialog  otype=sfix(16)  scale=2^-13  rndmethod=Biased  factor=1  satmethod=None  shift_vec=[0 1 2 -1]  value=round([0:255]/17)  inPortNames=[' '; ' ';]  outPortNames=[' '; 'c']  dspbaimage=dspba_prim_wide.svg  text=fprintf('convert');  style=Optimised  visibilities=8+64+256+2^17  clipdetect=off  floatPrecision=float32_m23  advOptions=[]  version=20211007
  Lut : DSPBAPrim/Lut  primtype=lut  nInputs=1  nOutputs=1  omode=Inherit via internal rule  otype=sfix(16)  scale=2^-15  rndmethod=Unbiased  factor=1  satmethod=Symmetric  shift_vec=[0 1 2 -1]  value=CPSample_Vector_LUT  inPortNames=[' '; ' ';]  outPortNames=[' ']  dspbaimage=dspba_prim.svg  text=fprintf('LUT');  style=Optimised  visibilities=8 + 1024  floatPrecision=float32_m23  version=20211007
  Lut1 : DSPBAPrim/Lut  primtype=lut  nInputs=1  nOutputs=1  omode=Inherit via internal rule  otype=sfix(16)  scale=2^-15  rndmethod=Unbiased  factor=1  satmethod=Symmetric  shift_vec=[0 1 2 -1]  value=Tsym_reinterpret_LUT  inPortNames=[' '; ' ';]  outPortNames=[' ']  dspbaimage=dspba_prim.svg  text=fprintf('LUT');  style=Optimised  visibilities=8 + 1024  floatPrecision=float32_m23  version=20211007
  Mult : DSPBAPrim/Mult  primtype=mult  nInputs=2  nOutputs=1  omode=Inherit via internal rule  otype=sfix(16)  scale=2^-15  rndmethod=Unbiased  factor=1  satmethod=Symmetric  shift_vec=[0 1 2 -1]  value=0  inPortNames=[' '; ' ';]  outPortNames=[' ']  dspbaimage=dspba_prim.svg  text=fprintf('X');  style=Optimised  visibilities=8+2^18+2^19  floatPrecision=float64_m52  floatRounding=correct  advOptions=[]  version=20211007
  Mult1 : DSPBAPrim/Mult  primtype=mult  nInputs=2  nOutputs=1  omode=Inherit via internal rule  otype=sfix(16)  scale=2^-15  rndmethod=Unbiased  factor=1  satmethod=Symmetric  shift_vec=[0 1 2 -1]  value=0  inPortNames=[' '; ' ';]  outPortNames=[' ']  dspbaimage=dspba_prim.svg  text=fprintf('X');  style=Optimised  visibilities=8+2^18+2^19  floatPrecision=float64_m52  floatRounding=correct  advOptions=[]  version=20211007
  Mux : DSPBAPrim/Mux  primtype=mux  nInputs=evalAionMaskParam(gcb,'value',1)+1  nOutputs=1  omode=Inherit via internal rule  otype=sfix(16)  scale=2^-15  rndmethod=Unbiased  factor=1  satmethod=Symmetric  shift_vec=[0 1 2 -1]  value=2  inPortNames=['s '; 'd0'; 'd1'; 'd2'; 'd3'; 'd4'; 'd5'; 'd6'; 'd7'; 'd8'; 'd9';]  outPortNames=[' ']  dspbaimage=dspba_prim_tall.svg  text=fprintf('%s', primtype);  style=Optimised  visibilities=1032  version=20211007
  Mux1 : DSPBAPrim/Mux  primtype=mux  nInputs=evalAionMaskParam(gcb,'value',1)+1  nOutputs=1  omode=Inherit via internal rule  otype=sfix(16)  scale=2^-15  rndmethod=Unbiased  factor=1  satmethod=Symmetric  shift_vec=[0 1 2 -1]  value=2  inPortNames=['s '; 'd0'; 'd1'; 'd2'; 'd3'; 'd4'; 'd5'; 'd6'; 'd7'; 'd8'; 'd9';]  outPortNames=[' ']  dspbaimage=dspba_prim_tall.svg  text=fprintf('%s', primtype);  style=Optimised  visibilities=1032  version=20211007
  Mux2 : DSPBAPrim/Mux  primtype=mux  nInputs=evalAionMaskParam(gcb,'value',1)+1  nOutputs=1  omode=Specify via dialog  otype=sfix(18)  scale=2^-15  rndmethod=Unbiased  factor=1  satmethod=Symmetric  shift_vec=[0 1 2 -1]  value=2  inPortNames=['s '; 'd0'; 'd1'; 'd2'; 'd3'; 'd4'; 'd5'; 'd6'; 'd7'; 'd8'; 'd9';]  outPortNames=[' ']  dspbaimage=dspba_prim_tall.svg  text=fprintf('%s', primtype);  style=Optimised  visibilities=1032  version=20211007
  Negate : DSPBAPrim/Negate  primtype=negate  nInputs=1  nOutputs=1  omode=Inherit via internal rule  otype=sfix(16)  scale=2^-15  rndmethod=Unbiased  factor=1  satmethod=Symmetric  shift_vec=[0 1 2 -1]  value=0  inPortNames=[' '; ' ';]  outPortNames=[' ']  dspbaimage=dspba_prim.svg  text=fprintf('-x');  style=Optimised  visibilities=8  version=20211007
  RegField1 : DSPBAModelBus/RegField  reg_name=4  reg_rwmode=Read/Write  reg_msb=31  reg_lsb=0  reg_mode=Specify via dialog  reg_type=ufix(32)  reg_scale=2^0  reg_init=F1_MSB  reg_desc="32 bit  of Carrier Center Frequency"  reg_modal=off  reg_desc0=0  reg_desc1=0  reg_desc2=0  reg_desc3=0  reg_desc4=0  reg_desc5=0  reg_desc6=0  reg_desc7=0  reg_addr=4  SampleTime=-1  version=20090407
  RegField2 : DSPBAModelBus/RegField  reg_name=reg_mem_offset_Phase_comp_enable  reg_rwmode=Read/Write  reg_msb=0  reg_lsb=0  reg_mode=Specify via dialog  reg_type=ufix(1)  reg_scale=2^0  reg_init=1  reg_desc=Enable/Disable Phase Compensation  reg_modal=off  reg_desc0=0  reg_desc1=0  reg_desc2=0  reg_desc3=0  reg_desc4=0  reg_desc5=0  reg_desc6=0  reg_desc7=0  reg_addr=1  SampleTime=-1  version=20090407
  RegField3 : DSPBAModelBus/RegField  reg_name=0  reg_rwmode=Read/Write  reg_msb=31  reg_lsb=0  reg_mode=Specify via dialog  reg_type=ufix(32)  reg_scale=2^0  reg_init=F1_LSB  reg_desc="32 bit  of Carrier Center Frequency LSB"  reg_modal=off  reg_desc0=0  reg_desc1=0  reg_desc2=0  reg_desc3=0  reg_desc4=0  reg_desc5=0  reg_desc6=0  reg_desc7=0  reg_addr=0  SampleTime=-1  version=20090407
  RegField4 : DSPBAModelBus/RegField  reg_name=reg_mem_offset_tx_rx_sel  reg_rwmode=Read/Write  reg_msb=0  reg_lsb=0  reg_mode=Specify via dialog  reg_type=ufix(1)  reg_scale=2^0  reg_init=PhaseGen_TXRX  reg_desc=Enable/Disable Phase Compensation  reg_modal=off  reg_desc0=0  reg_desc1=0  reg_desc2=0  reg_desc3=0  reg_desc4=0  reg_desc5=0  reg_desc6=0  reg_desc7=0  reg_addr=2  SampleTime=-1  version=20090407
  Sub : DSPBAPrim/Sub  primtype=sub  nInputs=2  nOutputs=1  omode=Inherit via internal rule with word growth  otype=sfix(16)  scale=2^-15  rndmethod=Unbiased  factor=1  satmethod=Symmetric  shift_vec=[0 1 2 -1]  value=0  inPortNames=['+'; '-';]  outPortNames=[' ']  dspbaimage=dspba_prim.svg  text=fprintf('-');  style=Optimised  visibilities=8+2^17+2^18  floatRounding=correct  advOptions=[]  version=20211007
  SynthesisInfo : DSPBAPrim/SynthesisInfo  primtype=synthinfo  nInputs=0  nOutputs=0  omode=Inherit via internal rule  otype=sfix(16)  scale=2^-15  rndmethod=Truncate  factor=1  satmethod=Symmetric  shift_vec=[0 1 2 -1]  value=99  inPortNames=[' '; ' ';]  outPortNames=[' ']  dspbaimage=dspba_prim_ctrl.jpg  text=fprintf('Style=%s', style);  style=Scheduled  visibilities=2^17+2^18+2^19+2^20+2^21+2^22+2^23+2^24  constraintPair=None  constraintRelation=>  constraintLimit=2  modelRefSign=+  modelRef=''  showSchedule=off  simulationMode=Use Global Value  resetMinimization=Conditional - On for ChannelIn/Out only  version=20220106
  Terminator : Terminator
  Terminator1 : Terminator
  Terminator2 : Terminator
  To Workspace : ToWorkspace  Commented=on  VariableName=F1_LO  SampleTime=-1
  To Workspace1 : ToWorkspace  Commented=on  VariableName=F1_HI  SampleTime=-1
  To Workspace2 : ToWorkspace  Commented=on  VariableName=F1_full  SampleTime=-1
  dout1 : Outport
  vout : Outport  Port=2
  cout : Outport  Port=3
  sin : Outport  Port=4
  cos : Outport  Port=5
  fft_size_out : Outport  Port=6
  CPLenout : Outport  Port=7
  nsc_out : Outport  Port=8
  eAxC_out : Outport  Port=9
  sym_metadata_out : Outport  Port=10
  ul_timeref_out : Outport  Port=11
  wires:
  c/1 -> ChannelIn/2
  ChannelIn/1 -> ChannelOut/1
  ChannelIn/2 -> Lut1/1, ChannelOut/2
  v/1 -> ChannelIn/1
  ChannelIn/3 -> ChannelOut/3
  d1/1 -> ChannelIn/3
  ChannelOut/1 -> vout/1
  ChannelOut/2 -> cout/1
  ChannelOut/3 -> dout1/1
  ChannelOut/4 -> sin/1
  ChannelIn/5 -> Lut/1
  Convert3/1 -> Mult1/1
  Mult1/1 -> Sub/1, Mux/2, CmpGE/1
  Const1/1 -> CmpGE/2
  CmpGE/1 -> Mux/1
  Sub/1 -> Mux/3
  Const2/1 -> Sub/2
  Const3/1 -> CORDIC/4
  Const4/1 -> CORDIC/1
  Const5/1 -> CORDIC/2
  CORDIC/3 -> Terminator1/1
  Convert5/1 -> CORDIC/3
  ChannelOut/5 -> cos/1
  RegField2/1 -> And/1
  Const7/1 -> Mux1/2
  CORDIC/1 -> ChannelOut/5
  Mux1/1 -> Convert5/1
  Lut/1 -> Convert4/1
  Mult/1 -> Convert3/1
  Mux/1 -> Mux1/3
  Convert4/1 -> Terminator2/1
  ChannelIn/6 -> ChooseBits/1
  And/1 -> Mux1/1
  ChooseBits/1 -> And/2
  Tsym1/1 -> ChannelIn/4
  cp_T1/1 -> ChannelIn/5
  CP_EN1/1 -> ChannelIn/6
  fft_size/1 -> ChannelIn/7
  CPLen/1 -> ChannelIn/8
  nsc/1 -> ChannelIn/9
  ChannelOut/6 -> fft_size_out/1
  ChannelOut/7 -> CPLenout/1
  ChannelOut/8 -> nsc_out/1
  ChannelIn/7 -> ChannelOut/6
  ChannelIn/8 -> ChannelOut/7
  ChannelIn/9 -> ChannelOut/8
  ChannelIn/4 -> Terminator/1
  Mux2/1 -> ChannelOut/4
  CORDIC/2 -> Negate/1, Mux2/2
  Negate/1 -> Mux2/3
  RegField4/1 -> Mux2/1
  Convert1/1 -> Mult/2
  Lut1/1 -> Mult/1
  Const6/1 -> Mult1/2
  ChannelIn/10 -> ChannelOut/9
  ChannelIn/11 -> ChannelOut/10
  eAxC/1 -> ChannelIn/10
  sym_metadata/1 -> ChannelIn/11
  ChannelOut/9 -> eAxC_out/1
  ChannelOut/10 -> sym_metadata_out/1
  ul_timerefin/1 -> ChannelIn/12
  ChannelIn/12 -> ChannelOut/11
  ChannelOut/11 -> ul_timeref_out/1
  RegField1/1 -> BitCombine/2
  RegField3/1 -> BitCombine/1
  BitCombine/1 -> Convert1/1
